simulink model "simulacion"  (R2017a)
settings: Solver=VariableStepAuto  StartTime=0.0  StopTime=10  RelTol=1e-3
settings Model: Creator=Manuel Mollon  LastModifiedBy=Manuel Mollon

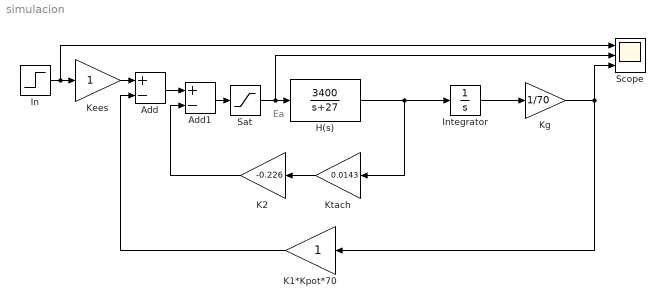
== system simulacion ==
  note: Ea
  Add : Sum  Inputs=+-
  Add1 : Sum  Inputs=+-
  H(s) : TransferFcn  Numerator=[3400]  Denominator=[1 27]
  In : Step  After=10  SampleTime=0
  Integrator : Integrator
  K1*Kpot*70 : Gain
  K2 : Gain  Gain=-0.226
  Kees : Gain
  Kg : Gain  Gain=1/70
  Ktach : Gain  Gain=0.0143
  Sat : Saturate  UpperLimit=6  LowerLimit=-6
  Scope : Scope  NumInputPorts=3
  wires:
  Add/1 -> Add1/1
  H(s)/1 -> Ktach/1, Integrator/1
  Kg/1 -> K1*Kpot*70/1, Scope/3
  K2/1 -> Add1/2
  K1*Kpot*70/1 -> Add/2
  In/1 -> Scope/1, Kees/1
  Integrator/1 -> Kg/1
  Ktach/1 -> K2/1
  Kees/1 -> Add/1
  Add1/1 -> Sat/1
  Sat/1 -> Scope/2, H(s)/1
